simulink model "Mechanical"  (R2022b)
settings: Solver=VariableStepAuto  StartTime=0.0  StopTime=10.0  RelTol=1e-3
settings Model: Creator=mliu  LastModifiedBy=mliu

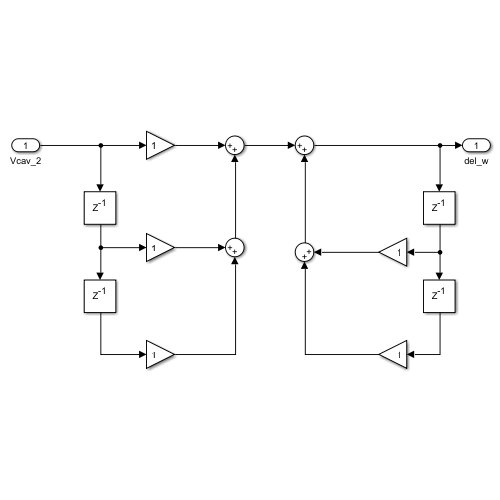
[thumbnail: Simulink's stored preview of the top-level diagram]
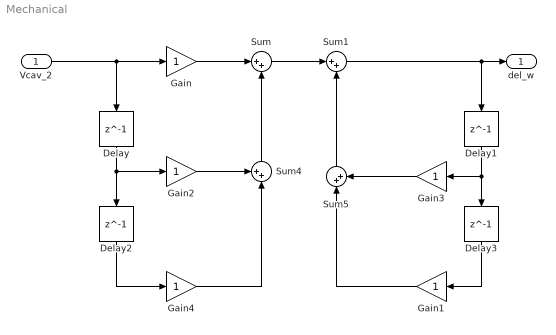
== system Mechanical ==
  Vcav_2 : Inport
  Delay{,1..3} (4 alike) : Delay  DelayLength=1  InitialCondition=0
  Gain{,1..4} (5 alike) : Gain
  Sum : Sum  Inputs=|++
  Sum1 : Sum  Inputs=|++
  Sum4 : Sum  Inputs=++|
  Sum5 : Sum  Inputs=|++
  del_w : Outport
  wires:
  Vcav_2/1 -> Delay/1, Gain/1
  Gain/1 -> Sum/1
  Sum/1 -> Sum1/1
  Sum1/1 -> Delay1/1, del_w/1
  Delay1/1 -> Gain3/1, Delay3/1
  Delay3/1 -> Gain1/1
  Gain1/1 -> Sum5/1
  Gain3/1 -> Sum5/2
  Sum5/1 -> Sum1/2
  Delay/1 -> Gain2/1, Delay2/1
  Delay2/1 -> Gain4/1
  Gain2/1 -> Sum4/1
  Gain4/1 -> Sum4/2
  Sum4/1 -> Sum/2
